simulink model "FK_IK"  (R2021a)
settings: Solver=VariableStepAuto  StartTime=0.0  StopTime=10  RelTol=1e-3
values from neighbouring files (symbols this model uses):
  adMotorLimits = [ 0, 180 ... (first row only)    [initSim.m]
libraries: robotcorelib x3, vrlib x3, robotmaniplib x2
settings Model: Creator=loris  LastModifiedBy=angelo

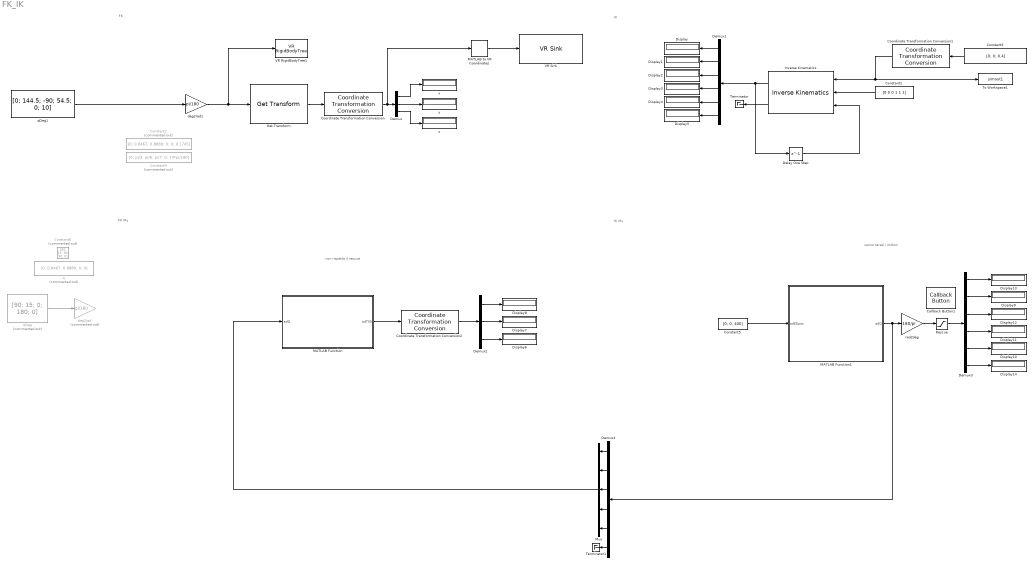
== system FK_IK ==
  note: non rispetta il rescue
  note: vanno tarati i motori
  note: IK My
  note: FK My
  note: FK
  note: IK
  Callback Button1 : CallbackButton  ButtonText=load motor limits
      settings: ClickFcn=|
      | % Motor Limits
      | adMotorLimits = [ 0, 180;
      |                  15, 165;
      |                   0, 180;
      |                   0, 180;
      |                   0, 180;
      |                  10,  73;
      | ];
  Constant1 : Constant  Value=[0 0 0 1 1 1]  VectorParams1D=off
  Constant2 : Constant  Commented=on  Value=[0; 0.8467; 0.8889; 0; 0; 0.1745]
  Constant3 : Constant  Value=[0; 0; 0.4]
  Constant4 : Constant  Commented=on  Value=[0; pi/3; pi/6; pi/7; 0; 73*pi/180]
  Constant5 : Constant  Value=[0; 0; 400]
  Constant6 : Constant  Commented=on  Value=[90; 15; 90; 90; 0]
  Coordinate Transformation Conversion : robotcorelib/Coordinate Transformation Conversion  InputRepresentation=Homogeneous Transformation  InputEulerSequence=ZYX  ShowTrVecInputPort=on  OutputRepresentation=Translation Vector  OutputEulerSequence=ZYX  ShowTrVecOutputPort=on  SimulateUsing=Code generation
      settings: SourceProductBaseCode=NV,RO,RR,UV
  Coordinate Transformation Conversion1 : robotcorelib/Coordinate Transformation Conversion  InputRepresentation=Translation Vector  InputEulerSequence=ZYX  ShowTrVecInputPort=on  OutputRepresentation=Homogeneous Transformation  OutputEulerSequence=ZYX  ShowTrVecOutputPort=on  SimulateUsing=Interpreted execution
      settings: SourceProductBaseCode=NV,RO,RR,UV
  Coordinate Transformation Conversion2 : robotcorelib/Coordinate Transformation Conversion  InputRepresentation=Homogeneous Transformation  InputEulerSequence=ZYX  ShowTrVecInputPort=on  OutputRepresentation=Translation Vector  OutputEulerSequence=ZYX  ShowTrVecOutputPort=on  SimulateUsing=Interpreted execution
      settings: SourceProductBaseCode=NV,RO,RR,UV
  Delay One Step : Delay  DelayLength=1  InitialCondition=zeros(6,1)
  Demux : Demux  Outputs=3
  Demux1 : Demux  Outputs=6
  Demux2 : Demux  Outputs=3
  Demux3 : Demux  Outputs=6
  Demux4 : Demux  Outputs=6
  Display{,1..14} (15 alike) : Display
  Get Transform : robotmaniplib/Get Transform  RigidBodyTree=oBraccio6dofee  SourceBody=ee  TargetBody=base_link  SimulateUsing=Interpreted execution
  Inverse Kinematics : robotmaniplib/Inverse Kinematics  RigidBodyTree=oBraccio6dofee  EndEffector=ee  ShowInfo=on  SolverName=BFGS Gradient Projection  EnforceJointLimits=on  MaxIterations=1500  MaxTime=10  GradientTolerance=1e-7  SolutionTolerance=1e-6  StepTolerance=1e-14  ErrorChangeTolerance=1e-12  UseErrorDamping=on  DampingBias=0.0025  SimulateUsing=Interpreted execution
  MATLAB Function : MATLAB Function  TreatAsAtomicUnit=on
  MATLAB Function1 : MATLAB Function  TreatAsAtomicUnit=on
  MATLAB to VR Coordinates : vrlib/Utilities/MATLAB to VR Coordinates
      settings: SourceProductBaseCode=SL
  Mux : Mux  Inputs=5
  Rescue : Saturate  UpperLimit=adMotorLimits(:,2)  LowerLimit=adMotorLimits(:,1)
  Terminator : Terminator
  Terminator1 : Terminator
  To Workspace1 : ToWorkspace  VariableName=simout1  SaveFormat=Structure  SampleTime=-1
  VR RigidBodyTree1 : vrlib/VR RigidBodyTree  VrmlFile=/home/angelo/1.PROJECTS/arm-manipulator-6dof/Foo/robotWorld.x3d  RBT=oBraccio6dofee  useRBT=off  Ts=-1  ForceViewerOpen=off
      settings: SourceProductBaseCode=SL
  VR Sink : vrlib/VR Sink  InstantiateOnLoad=on  SampleTime=0.1  ViewEnable=on  RemoteChange=off  RemoteView=off  FieldsWritten=SetPoint.translation.3.1.1.double  WorldFileName=Foo/robotWorld.x3d  WorldDescription=Simple Robot Scene  AutoView=off  VideoDimensions=[]  AllowVariableSize=off
  deg2rad : Gain  Commented=on  Gain=pi/180
  deg2rad1 : Gain  Gain=pi/180
  q : Constant  Commented=on  Value=[0; 0.8467; 0.8889; 0; 0]
  qDeg : Constant  Commented=on  Value=[90; 15; 0; 180; 0]
  qDeg1 : Constant  Value=[0; 144.5; -90; 54.5; 0; 10]
  rad2deg : Gain  Gain=180/pi
  x : Display
  y : Display
  z : Display
  wires:
  Get Transform/1 -> Coordinate Transformation Conversion/1
  Coordinate Transformation Conversion/1 -> MATLAB to VR Coordinates/1, Demux/1
  Demux/1 -> x/1
  Demux/2 -> y/1
  Demux/3 -> z/1
  Constant1/1 -> Inverse Kinematics/2
  Inverse Kinematics/1 -> Demux1/1, Delay One Step/1
  Inverse Kinematics/2 -> Terminator/1
  Demux1/1 -> Display/1
  Demux1/2 -> Display1/1
  Demux1/3 -> Display2/1
  Demux1/4 -> Display3/1
  Demux1/5 -> Display4/1
  Demux1/6 -> Display5/1
  Constant3/1 -> Coordinate Transformation Conversion1/1
  Coordinate Transformation Conversion1/1 -> Inverse Kinematics/1, To Workspace1/1
  Delay One Step/1 -> Inverse Kinematics/3
  MATLAB to VR Coordinates/1 -> VR Sink/1
  MATLAB Function/1(adT05) -> Coordinate Transformation Conversion2/1
  Coordinate Transformation Conversion2/1 -> Demux2/1
  Demux2/1 -> Display8/1
  Demux2/2 -> Display7/1
  Demux2/3 -> Display6/1
  deg2rad1/1 -> VR RigidBodyTree1/1, Get Transform/1
  qDeg1/1 -> deg2rad1/1
  MATLAB Function1/1(adQ) -> Demux4/1, rad2deg/1
  Demux3/1 -> Display13/1
  Demux3/2 -> Display9/1
  Demux3/3 -> Display12/1
  Demux3/4 -> Display11/1
  Demux3/5 -> Display10/1
  Demux3/6 -> Display14/1
  Constant5/1 -> MATLAB Function1/1(adEEpos)
  Rescue/1 -> Demux3/1
  rad2deg/1 -> Rescue/1
  qDeg/1 -> deg2rad/1
  Demux4/2 -> Mux/2
  Demux4/1 -> Mux/1
  Demux4/3 -> Mux/3
  Demux4/4 -> Mux/4
  Demux4/5 -> Mux/5
  Demux4/6 -> Terminator1/1
  Mux/1 -> MATLAB Function/1(adQ)

== matlab function FK_IK/MATLAB Function1 ==
  data: adEEpos input; adQ output
function adQ = IKIN(adEEpos)
%{
    @param      adEEpos:    (x; y; z;) desired EE position.
    @return     adQ:        Joints configuration (6, 1).
%}

% DH parameter
dh      = load('data/dhBraccioParam.mat');

% Motors mapping
adJc    = fIKIN(adEEpos, dh.adD, dh.adA);
q1      = pi/2 - adJc(1);
q2      = adJc(2);
q3      = adJc(3) + pi/2;
q4      = adJc(4) + pi/2;
q5      = adJc(5);
q6      = 0;

% Output
adQ     = [q1; q2; q3; q4; q5; q6];

end

== matlab function FK_IK/MATLAB Function ==
  data: adT05 output; adQ input
function adT05  = KIN(adQ)
%{
    @param      adQ:        Joints configuration.
    @param      adOffset:   Offset to map motors.
    @return     T05:        Homogeneus Transformation Matrix.
%}

% DH parameter
dh      = load('data/dhBraccioParam.mat');

% Motors Mapping
q1      = (adQ(1) - pi/2) * -1;
q2      = adQ(2);
q3      = adQ(3) - pi/2;
q4      = adQ(4) - pi/2;
q5      = adQ(5);

% Joints configuration
adQ     = [q1; q2; q3; q4; q5];

% Output
adT05   = fKIN(dh.adD, adQ, dh.adA, dh.adAlpha);

end
